simulink model "homework5_sim"  (R2025b)
settings: Solver=VariableStepAuto  StartTime=0.0  StopTime=10.0  RelTol=1e-3
values from neighbouring files (symbols this model uses):
  A = readmatrix("yunzhuorui/GTIIT/2026-Spring/Control_theory/Homework/Homework4/HW4_A.xlsx")    [Homework5.m]
  B = [1;0;2;0]    [Homework5.m]
  C = [0 1 0 3]    [Homework5.m]
  D = 0    [Homework5.m]
  K = [14.594417419680658, 0.999096975937301, -1.297208709840328, 9.145289774526315]    [Homework5.m]
  L = acker(A', C', est_poles)'    [Homework5.m]
  Nbar = Nu + K * Nx    [Homework5.m]
settings Model: Creator=yunzhuorui  LastModifiedBy=yunzhuorui

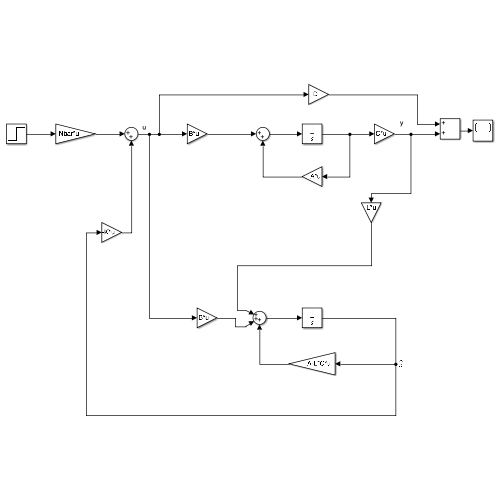
[thumbnail: Simulink's stored preview of the top-level diagram]
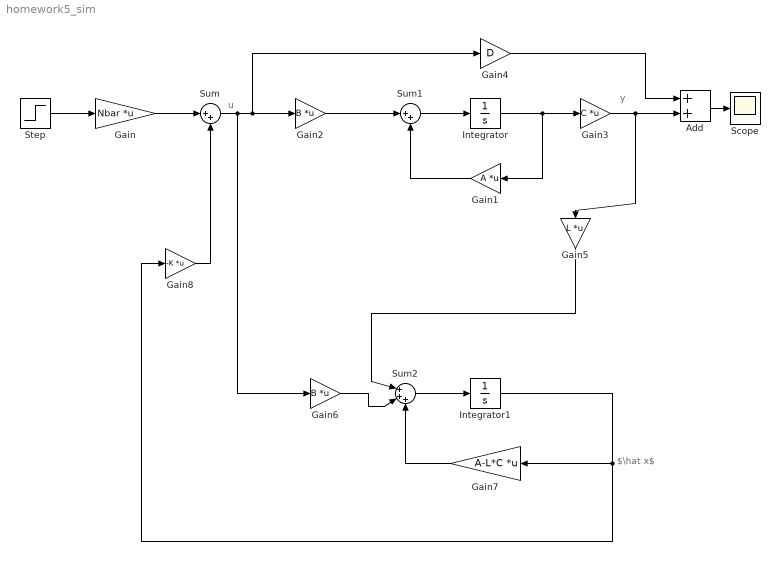
== system homework5_sim ==
  note: $\hat x$
  note: y
  note: u
  Add : Sum
  Gain : Gain  Gain=Nbar  Multiplication=Matrix(K*u)
  Gain1 : Gain  Gain=A  Multiplication=Matrix(K*u)
  Gain2 : Gain  Gain=B  Multiplication=Matrix(K*u)
  Gain3 : Gain  Gain=C  Multiplication=Matrix(K*u)
  Gain4 : Gain  Gain=D
  Gain5 : Gain  Gain=L  Multiplication=Matrix(K*u)
  Gain6 : Gain  Gain=B  Multiplication=Matrix(K*u)
  Gain7 : Gain  Gain=A-L*C  Multiplication=Matrix(K*u)
  Gain8 : Gain  Gain=-K  Multiplication=Matrix(K*u)
  Integrator : Integrator
  Integrator1 : Integrator
  Scope : Scope
      settings: ActiveDisplayYMinimum=1.0065318038934983  ActiveDisplayYMaximum=1.007301819116224
  Step : Step  SampleTime=0
  Sum : Sum  Inputs=|++
  Sum1 : Sum  Inputs=|++
  Sum2 : Sum  Inputs=|+++
  wires:
  Step/1 -> Gain/1
  Gain/1 -> Sum/1
  Sum/1 -> Gain6/1, Gain4/1, Gain2/1
  Gain2/1 -> Sum1/1
  Sum1/1 -> Integrator/1
  Integrator/1 -> Gain1/1, Gain3/1
  Gain1/1 -> Sum1/2
  Gain4/1 -> Add/1
  Add/1 -> Scope/1
  Gain6/1 -> Sum2/2
  Gain3/1 -> Gain5/1, Add/2
  Gain5/1 -> Sum2/1
  Sum2/1 -> Integrator1/1
  Integrator1/1 -> Gain7/1, Gain8/1
  Gain7/1 -> Sum2/3
  Gain8/1 -> Sum/2
